simulink model "HFI_Simulink"  (R2023a)
settings: Solver=FixedStepAuto  StartTime=0.0  StopTime=10.0  FixedStep=1e-4  RelTol=1e-3
model workspace (MAT data in the model file):
  cntPRD = Simulink.Parameter
  cntPRD.Value = 30
  cntPRD.DataType = 'uint16'
  cntPRD.Complexity = 'real'
  cntPRD.Dimensions = [1 1]
undefined symbols (not defined in the file): HFI_Status
libraries: simulink x4
settings Model: DataDictionary=HFI_Merge.sldd  Creator=洲  LastModifiedBy=洲
settings OptimizationCC: DefaultParameterBehavior=Inlined  EnhancedBackFolding=on  PassReuseOutputArgsAs=Individual arguments  ZeroExternalMemoryAtStartup=off  ZeroInternalMemoryAtStartup=off  OptimizeBlockOrder=speed  DifferentSizesBufferReuse=on  OptimizationCustomize=off  EfficientTunableParamExpr=on
settings DebuggingCC: ParameterTunabilityLossMsg=error
settings SFSimCC: MATLABDynamicMemAlloc=off
settings RTWCC: Description=Embedded Coder  SystemTargetFile=ert.tlc  TemplateMakefile=ert_default_tmf
settings CodeAppCC: ForceParamTrailComments=on  IgnoreCustomStorageClasses=off  OperatorAnnotations=on  SimulinkDataObjDesc=on  SFDataObjDesc=on  InsertBlockDesc=on
settings ERTTargetCC: TargetLangStandard=C99 (ISO)  GenerateSampleERTMain=on  InlinedParameterPlacement=NonHierarchical  ERTCustomFileTemplate=example_file_process.tlc

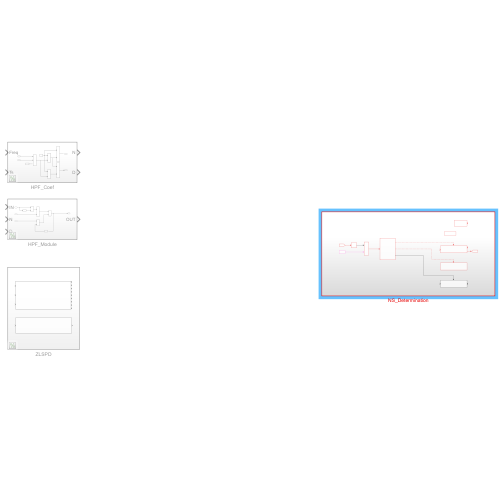
[thumbnail: Simulink's stored preview of the top-level diagram]
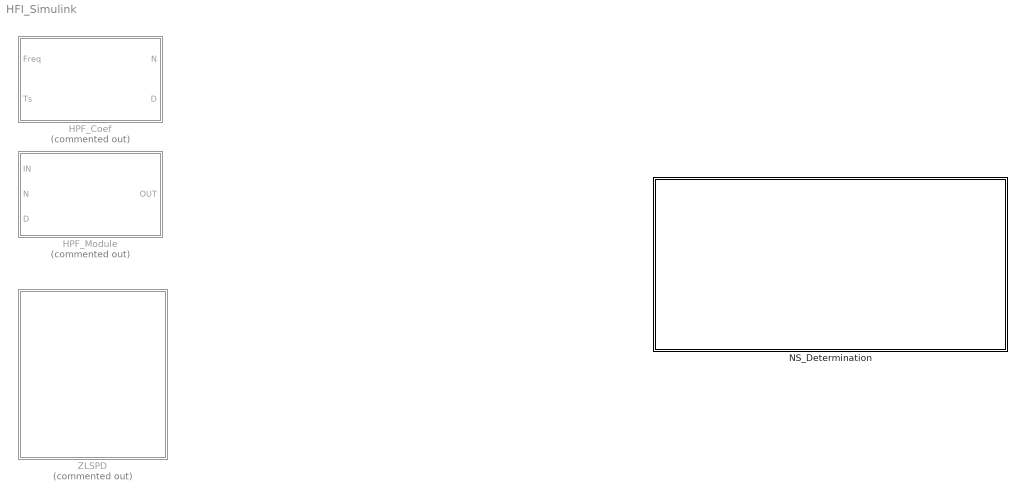
== system HFI_Simulink ==
  HPF_Coef : Subsystem  Commented=on
  HPF_Module : Subsystem  Commented=on
  NS_Determination : Subsystem
  ZLSPD : Subsystem  Commented=on

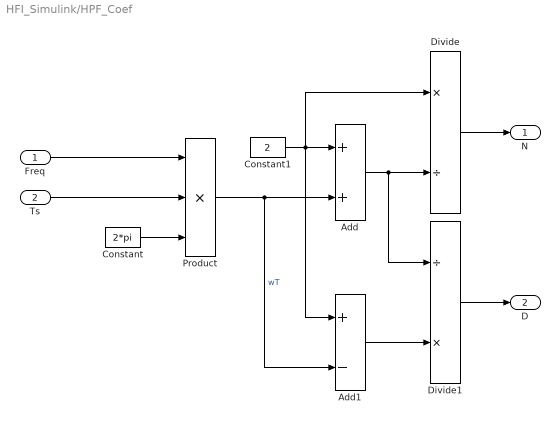
== system HFI_Simulink/HPF_Coef ==
  Freq : Inport
  Ts : Inport  Port=2
  Add : Sum
  Add1 : Sum  Inputs=+-
  Constant : Constant  Value=2*pi  OutDataTypeStr=single
  Constant1 : Constant  Value=2  OutDataTypeStr=single
  Divide : Product  Inputs=*/
  Divide1 : Product  Inputs=/*
  Product : Product  Inputs=3
  N : Outport
  D : Outport  Port=2
  wires:
  Freq/1 -> Product/1
  Constant/1 -> Product/3
  Ts/1 -> Product/2
  Add/1 -> Divide1/1, Divide/2
  Product/1 -> Add1/2, Add/2  "wT"
  Constant1/1 -> Add/1, Divide/1, Add1/1
  Divide/1 -> N/1
  Add1/1 -> Divide1/2
  Divide1/1 -> D/1

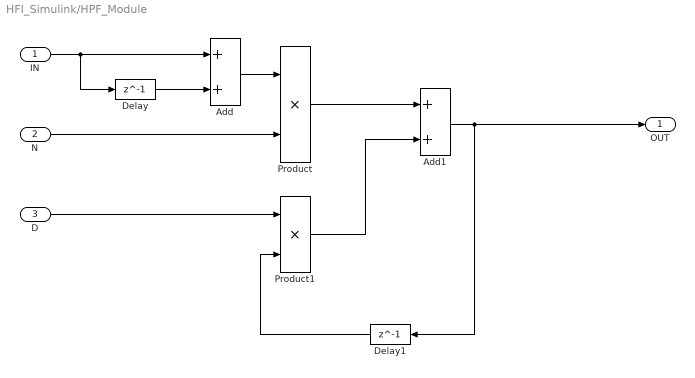
== system HFI_Simulink/HPF_Module ==
  IN : Inport
  N : Inport  Port=2
  D : Inport  Port=3
  Add : Sum
  Add1 : Sum
  Delay : Delay  DelayLength=1
  Delay1 : Delay  DelayLength=1
  Product : Product
  Product1 : Product
  OUT : Outport
  wires:
  IN/1 -> Delay/1, Add/1
  Delay/1 -> Add/2
  Add/1 -> Product/1
  N/1 -> Product/2
  Product/1 -> Add1/1
  D/1 -> Product1/1
  Add1/1 -> OUT/1, Delay1/1
  Delay1/1 -> Product1/2
  Product1/1 -> Add1/2

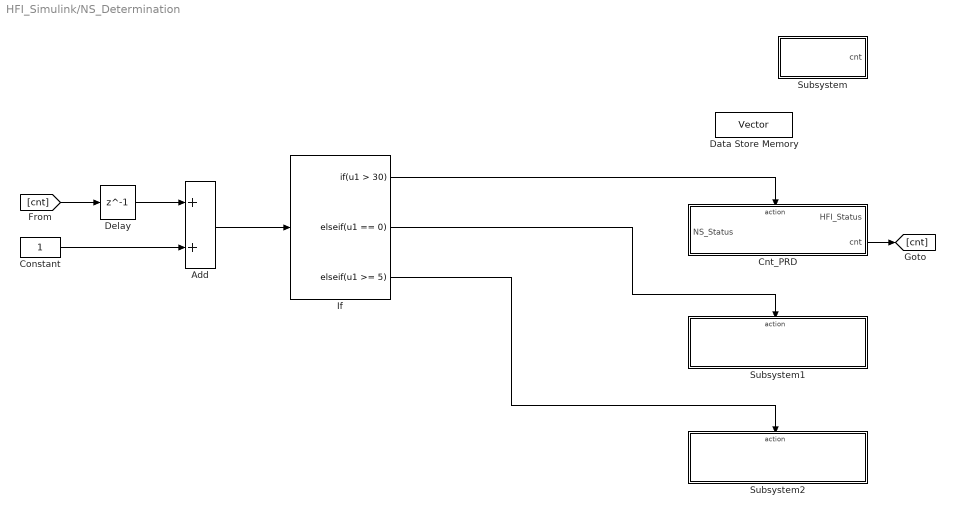
== system HFI_Simulink/NS_Determination ==
  Add : Sum
  Cnt_PRD : Subsystem  TreatAsAtomicUnit=on
  Constant : Constant  OutDataTypeStr=uint16
  Data Store Memory : DataStoreMemory  DataStoreName=Vector  WriteAfterWriteMsg=warning  ShowAdditionalParam=off
  Delay : Delay  DelayLength=1
  If : If  IfExpression=u1 > 30  ElseIfExpressions=u1 == 0,u1 >= 5  ShowElse=off
  Subsystem : Subsystem
  Subsystem1 : Subsystem
  Subsystem2 : Subsystem
  wires:
  If/1 -> Cnt_PRD/Action
  Constant/1 -> Add/2
  Add/1 -> If/1
  Cnt_PRD/2(cnt) -> [cnt]
  [cnt] -> Delay/1
  If/2 -> Subsystem1/Action
  Delay/1 -> Add/1
  If/3 -> Subsystem2/Action

== system HFI_Simulink/ZLSPD ==
  HFI_NSID_STATE : Subsystem
  HFI_RESET_STATE : Subsystem

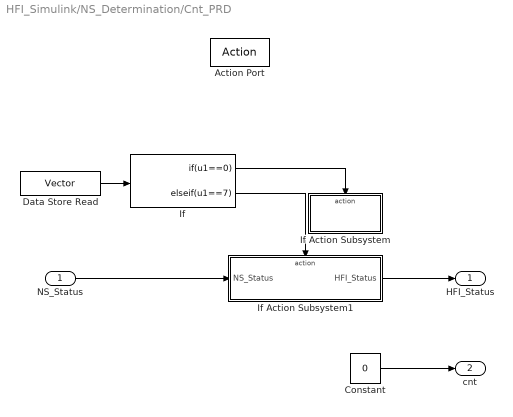
== system HFI_Simulink/NS_Determination/Cnt_PRD ==
  NS_Status : Inport
  Action Port : ActionPort  ActionPortLabel=if(u1 > 30)
  Constant : Constant  Value=0  OutDataTypeStr=uint16
  Data Store Read : DataStoreRead  DataStoreName=Vector  IndexOptions=Index vector (dialog)  Indices=1  OutputSizes=1
  If : If  IfExpression=u1==0  ElseIfExpressions=u1==7  ShowElse=off
  If Action Subsystem : Subsystem  TreatAsAtomicUnit=on
  If Action Subsystem1 : Subsystem  TreatAsAtomicUnit=on
  HFI_Status : Outport
  cnt : Outport  Port=2
  wires:
  Data Store Read/1 -> If/1
  If/1 -> If Action Subsystem/Action
  If/2 -> If Action Subsystem1/Action
  If Action Subsystem1/1(HFI_Status) -> HFI_Status/1
  NS_Status/1 -> If Action Subsystem1/1(NS_Status)
  Constant/1 -> cnt/1

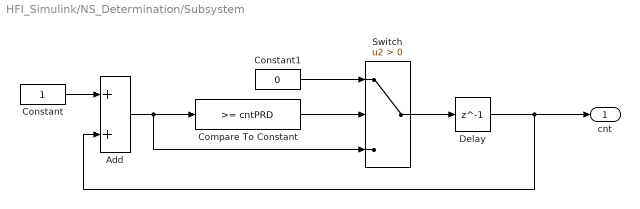
== system HFI_Simulink/NS_Determination/Subsystem ==
  Add : Sum
  Compare To Constant : simulink/Logic and Bit Operations/Compare To Constant  relop=>=  const=cntPRD  OutDataTypeStr=boolean
  Constant : Constant  OutDataTypeStr=uint16
  Constant1 : Constant  Value=0  OutDataTypeStr=uint16
  Delay : Delay  DelayLength=1
  Switch : Switch  Criteria=u2 > Threshold  SaturateOnIntegerOverflow=off  InputSameDT=off
  cnt : Outport
  wires:
  Constant1/1 -> Switch/1
  Compare To Constant/1 -> Switch/2
  Switch/1 -> Delay/1
  Add/1 -> Switch/3, Compare To Constant/1
  Delay/1 -> cnt/1, Add/2
  Constant/1 -> Add/1

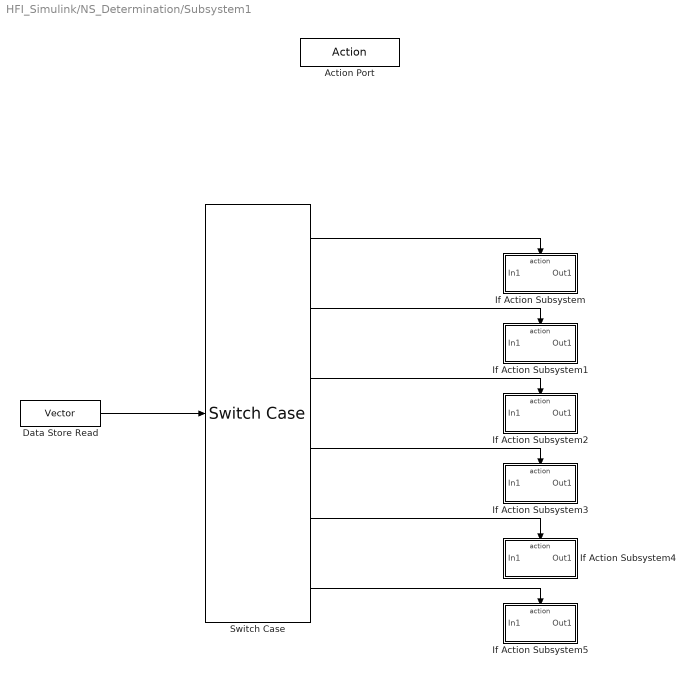
== system HFI_Simulink/NS_Determination/Subsystem1 ==
  Action Port : ActionPort  ActionPortLabel=elseif(u1 == 0)
  Data Store Read : DataStoreRead  DataStoreName=Vector  IndexOptions=Index vector (dialog)  Indices=1  OutputSizes=1
  If Action Subsystem : Subsystem  TreatAsAtomicUnit=on
  If Action Subsystem1 : Subsystem  TreatAsAtomicUnit=on
  If Action Subsystem2 : Subsystem  TreatAsAtomicUnit=on
  If Action Subsystem3 : Subsystem  TreatAsAtomicUnit=on
  If Action Subsystem4 : Subsystem  TreatAsAtomicUnit=on
  If Action Subsystem5 : Subsystem  TreatAsAtomicUnit=on
  Switch Case : SwitchCase  CaseConditions={1,2,3,4,5,6}  ShowDefaultCase=off
  wires:
  Data Store Read/1 -> Switch Case/1
  Switch Case/1 -> If Action Subsystem/Action
  Switch Case/2 -> If Action Subsystem1/Action
  Switch Case/3 -> If Action Subsystem2/Action
  Switch Case/4 -> If Action Subsystem3/Action
  Switch Case/5 -> If Action Subsystem4/Action
  Switch Case/6 -> If Action Subsystem5/Action

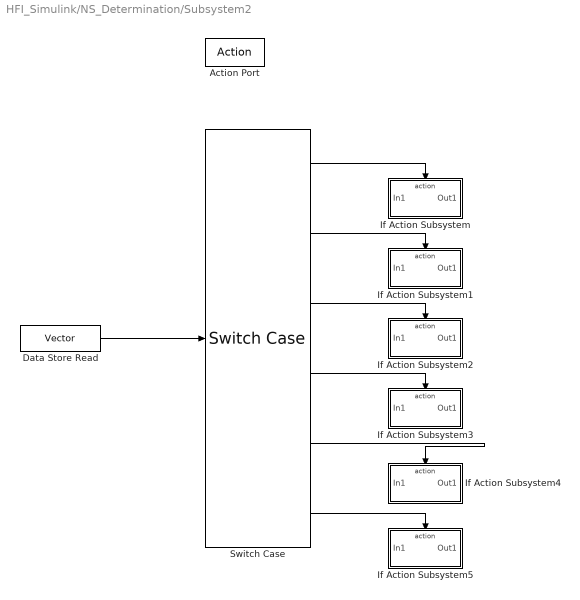
== system HFI_Simulink/NS_Determination/Subsystem2 ==
  Action Port : ActionPort  ActionPortLabel=elseif(u1 >= 5)
  Data Store Read : DataStoreRead  DataStoreName=Vector  IndexOptions=Index vector (dialog)  Indices=1  OutputSizes=1
  If Action Subsystem : Subsystem  TreatAsAtomicUnit=on
  If Action Subsystem1 : Subsystem  TreatAsAtomicUnit=on
  If Action Subsystem2 : Subsystem  TreatAsAtomicUnit=on
  If Action Subsystem3 : Subsystem  TreatAsAtomicUnit=on
  If Action Subsystem4 : Subsystem  TreatAsAtomicUnit=on
  If Action Subsystem5 : Subsystem  TreatAsAtomicUnit=on
  Switch Case : SwitchCase  CaseConditions={1,2,3,4,5,6}  ShowDefaultCase=off
  wires:
  Switch Case/5 -> If Action Subsystem4/Action
  Data Store Read/1 -> Switch Case/1
  Switch Case/3 -> If Action Subsystem2/Action
  Switch Case/4 -> If Action Subsystem3/Action
  Switch Case/1 -> If Action Subsystem/Action
  Switch Case/6 -> If Action Subsystem5/Action
  Switch Case/2 -> If Action Subsystem1/Action

== system HFI_Simulink/ZLSPD/HFI_NSID_STATE ==
  In1 : Inport
  Out1 : Outport
  wires:
  In1/1 -> Out1/1

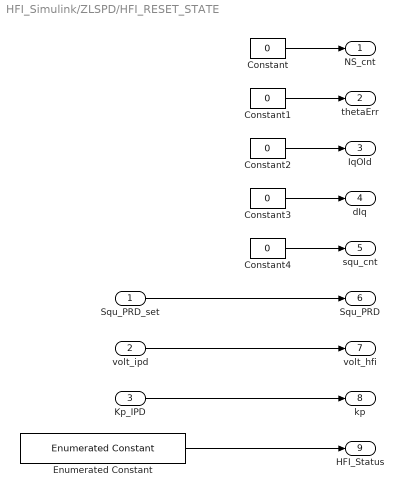
== system HFI_Simulink/ZLSPD/HFI_RESET_STATE ==
  Squ_PRD_set : Inport
  volt_ipd : Inport  Port=2
  Kp_IPD : Inport  Port=3
  Constant{,1..4} (5 alike) : Constant  Value=0  OutDataTypeStr=single
  Enumerated Constant : simulink/Sources/Enumerated Constant  OutDataTypeStr=Enum: HFI_Status  Value=HFI_Status.HFI_RESET_STATE  SampleTime=inf
  NS_cnt : Outport
  thetaErr : Outport  Port=2
  IqOld : Outport  Port=3
  dIq : Outport  Port=4
  squ_cnt : Outport  Port=5
  Squ_PRD : Outport  Port=6
  volt_hfi : Outport  Port=7
  kp : Outport  Port=8
  HFI_Status : Outport  Port=9
  wires:
  Constant/1 -> NS_cnt/1
  Constant1/1 -> thetaErr/1
  Constant2/1 -> IqOld/1
  Constant3/1 -> dIq/1
  Constant4/1 -> squ_cnt/1
  Squ_PRD_set/1 -> Squ_PRD/1
  volt_ipd/1 -> volt_hfi/1
  Kp_IPD/1 -> kp/1
  Enumerated Constant/1 -> HFI_Status/1

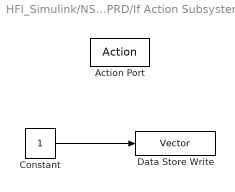
== system HFI_Simulink/NS_Determination/Cnt_PRD/If Action Subsystem ==
  Action Port : ActionPort  ActionPortLabel=if(u1==0)
  Constant : Constant  OutDataTypeStr=uint16
  Data Store Write : DataStoreWrite  DataStoreName=Vector  IndexOptions=Index vector (dialog)  Indices=1  OutputSizes=1
  wires:
  Constant/1 -> Data Store Write/1

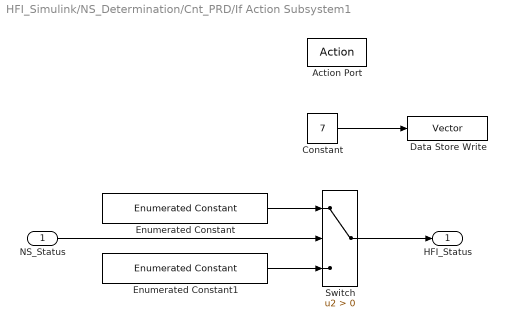
== system HFI_Simulink/NS_Determination/Cnt_PRD/If Action Subsystem1 ==
  NS_Status : Inport
  Action Port : ActionPort  ActionPortLabel=elseif(u1==7)
  Constant : Constant  Value=7  OutDataTypeStr=uint16
  Data Store Write : DataStoreWrite  DataStoreName=Vector  IndexOptions=Index vector (dialog)  Indices=1  OutputSizes=1
  Enumerated Constant : simulink/Sources/Enumerated Constant  OutDataTypeStr=Enum: HFI_Status  Value=HFI_Status.HFI_RUN_STATE  SampleTime=inf
  Enumerated Constant1 : simulink/Sources/Enumerated Constant  OutDataTypeStr=Enum: HFI_Status  Value=HFI_Status.HFI_RESET_STATE  SampleTime=inf
  Switch : Switch  Criteria=u2 > Threshold  SaturateOnIntegerOverflow=off  InputSameDT=off
  HFI_Status : Outport
  wires:
  Constant/1 -> Data Store Write/1
  NS_Status/1 -> Switch/2
  Enumerated Constant/1 -> Switch/1
  Enumerated Constant1/1 -> Switch/3
  Switch/1 -> HFI_Status/1

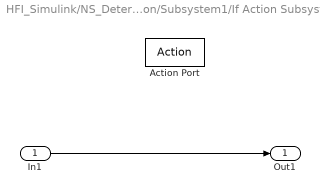
== system HFI_Simulink/NS_Determination/Subsystem1/If Action Subsystem ==
  In1 : Inport
  Action Port : ActionPort  ActionPortLabel=case [ 1 ]:
  Out1 : Outport
  wires:
  In1/1 -> Out1/1

== system HFI_Simulink/NS_Determination/Subsystem1/If Action Subsystem1 ==
  In1 : Inport
  Action Port : ActionPort  ActionPortLabel=case [ 2 ]:
  Out1 : Outport
  wires:
  In1/1 -> Out1/1

== system HFI_Simulink/NS_Determination/Subsystem1/If Action Subsystem2 ==
  In1 : Inport
  Action Port : ActionPort  ActionPortLabel=case [ 3 ]:
  Out1 : Outport
  wires:
  In1/1 -> Out1/1

== system HFI_Simulink/NS_Determination/Subsystem1/If Action Subsystem3 ==
  In1 : Inport
  Action Port : ActionPort  ActionPortLabel=case [ 4 ]:
  Out1 : Outport
  wires:
  In1/1 -> Out1/1

== system HFI_Simulink/NS_Determination/Subsystem1/If Action Subsystem4 ==
  In1 : Inport
  Action Port : ActionPort  ActionPortLabel=case [ 5 ]:
  Out1 : Outport
  wires:
  In1/1 -> Out1/1

== system HFI_Simulink/NS_Determination/Subsystem1/If Action Subsystem5 ==
  In1 : Inport
  Action Port : ActionPort  ActionPortLabel=case [ 6 ]:
  Out1 : Outport
  wires:
  In1/1 -> Out1/1

== system HFI_Simulink/NS_Determination/Subsystem2/If Action Subsystem ==
  In1 : Inport
  Action Port : ActionPort  ActionPortLabel=case [ 1 ]:
  Out1 : Outport
  wires:
  In1/1 -> Out1/1

== system HFI_Simulink/NS_Determination/Subsystem2/If Action Subsystem1 ==
  In1 : Inport
  Action Port : ActionPort  ActionPortLabel=case [ 2 ]:
  Out1 : Outport
  wires:
  In1/1 -> Out1/1

== system HFI_Simulink/NS_Determination/Subsystem2/If Action Subsystem2 ==
  In1 : Inport
  Action Port : ActionPort  ActionPortLabel=case [ 3 ]:
  Out1 : Outport
  wires:
  In1/1 -> Out1/1

== system HFI_Simulink/NS_Determination/Subsystem2/If Action Subsystem3 ==
  In1 : Inport
  Action Port : ActionPort  ActionPortLabel=case [ 4 ]:
  Out1 : Outport
  wires:
  In1/1 -> Out1/1

== system HFI_Simulink/NS_Determination/Subsystem2/If Action Subsystem4 ==
  In1 : Inport
  Action Port : ActionPort  ActionPortLabel=case [ 5 ]:
  Out1 : Outport
  wires:
  In1/1 -> Out1/1

== system HFI_Simulink/NS_Determination/Subsystem2/If Action Subsystem5 ==
  In1 : Inport
  Action Port : ActionPort  ActionPortLabel=case [ 6 ]:
  Out1 : Outport
  wires:
  In1/1 -> Out1/1
